simulink model "SF045A_HwAgSysArbn"  (R2013b)
settings: Solver=FixedStepDiscrete  SolverMode=SingleTasking  StartTime=0.0  StopTime=1  FixedStep=.002  RelTol=1e-3
values from neighbouring files (symbols this model uses):
  ARCHGLBPRM_2MILLISEC_SEC_F32 = DataDict.Constant    [SF045A_HwAgSysArbn_DataDict.m]
  ARCHGLBPRM_FLOATZEROTHD_ULS_F32 = DataDict.Constant    [SF045A_HwAgSysArbn_DataDict.m]
  ARCHGLBPRM_PIOVER180_ULS_F32 = DataDict.Constant    [SF045A_HwAgSysArbn_DataDict.m]
  CNVSECTOCNT_ULS_U32 = DataDict.Constant    [SF045A_HwAgSysArbn_DataDict.m]
  CNVTOMILLISEC_MILLISECPERCNT_F32 = DataDict.Constant    [SF045A_HwAgSysArbn_DataDict.m]
  FltInj_f32 = DataDict.Client    [SF045A_HwAgSysArbn_DataDict.m]
  FLTINJ_HWAGSYSARBN_HWAG = DataDict.Constant    [SF045A_HwAgSysArbn_DataDict.m]
  FLTINJ_HWAGSYSARBN_SERLCOMHWAG = DataDict.Constant    [SF045A_HwAgSysArbn_DataDict.m]
  HwAgCorrlnFlt = DataDict.NTC    [SF045A_HwAgSysArbn_DataDict.m]
  HwAgSnsrlsThdExcdd = DataDict.NTC    [SF045A_HwAgSysArbn_DataDict.m]
  HwAgSysArbnHwAgConf1Snsr = DataDict.Calibration    [SF045A_HwAgSysArbn_DataDict.m]
  HwAgSysArbnHwAgConf2Snsr = DataDict.Calibration    [SF045A_HwAgSysArbn_DataDict.m]
  HwAgSysArbnHwAgConfNoSnsr = DataDict.Calibration    [SF045A_HwAgSysArbn_DataDict.m]
  HwAgSysArbnHwAgCorrdCorrlnThd = DataDict.Calibration    [SF045A_HwAgSysArbn_DataDict.m]
  HwAgSysArbnHwAgCorrlnFailDebStep = DataDict.Calibration    [SF045A_HwAgSysArbn_DataDict.m]
  HwAgSysArbnHwAgCorrlnPassDebStep = DataDict.Calibration    [SF045A_HwAgSysArbn_DataDict.m]
  HwAgSysArbnHwAgCorrlnRng = DataDict.Calibration    [SF045A_HwAgSysArbn_DataDict.m]
  HwAgSysArbnHwAgSlewRate = DataDict.Calibration    [SF045A_HwAgSysArbn_DataDict.m]
  HwAgSysArbnHwAgSnsrlsCorrlnThd = DataDict.Calibration    [SF045A_HwAgSysArbn_DataDict.m]
  HwAgSysArbnHwAgSnsrlsKineThd = DataDict.Calibration    [SF045A_HwAgSysArbn_DataDict.m]
  HwAgSysArbnHwAgToMotAgCorrlnElpdTiLim = DataDict.Calibration    [SF045A_HwAgSysArbn_DataDict.m]
  HwAgSysArbnSerlComHwAgCorrdConf = DataDict.Calibration    [SF045A_HwAgSysArbn_DataDict.m]
  HwAgSysArbnSerlComHwAgSnsrlsConf = DataDict.Calibration    [SF045A_HwAgSysArbn_DataDict.m]
  HwAgSysArbnSlewRateTmr = DataDict.Calibration    [SF045A_HwAgSysArbn_DataDict.m]
  HWAGTHD_ULS_FLOAT32 = DataDict.Constant    [SF045A_HwAgSysArbn_DataDict.m]
  INVLDSRC_CNT_S08 = DataDict.Constant    [SF045A_HwAgSysArbn_DataDict.m]
  LRGSLEW_HWDEGPERSEC_F32 = DataDict.Constant    [SF045A_HwAgSysArbn_DataDict.m]
  NODEBSTEP_CNT_U16 = DataDict.Constant    [SF045A_HwAgSysArbn_DataDict.m]
  SLEWINPROGS_CNT_LGC = DataDict.Constant    [SF045A_HwAgSysArbn_DataDict.m]
  SLEWNOTINPROGS_CNT_LGC = DataDict.Constant    [SF045A_HwAgSysArbn_DataDict.m]
  SNSRDATASRCSELD_CNT_S08 = DataDict.Constant    [SF045A_HwAgSysArbn_DataDict.m]
  SNSRLSDATASRCSELD_CNT_S08 = DataDict.Constant    [SF045A_HwAgSysArbn_DataDict.m]
  SysGlbPrmSysKineRat = DataDict.ImprtdCal    [SF045A_HwAgSysArbn_DataDict.m]
  SysGlbPrmTorsBarStfn = DataDict.ImprtdCal    [SF045A_HwAgSysArbn_DataDict.m]
  ZEROTMR_MILLISEC_F32 = DataDict.Constant    [SF045A_HwAgSysArbn_DataDict.m]
undefined symbols (not defined in the file or in its folder): NtcSts1
libraries: NxtrLim x11, simulink x6, NxtrAbslt x6, Fil x3, autosarlib x2
(part 5 of 6)

== system SF045A_HwAgSysArbn/HwAgSysArbn/HwAgSysArbnPer1/HwAgArbn/CalcPinionVel/PinionAnglegConf/HwAg_Derivative ==
  HwAg : Inport
  Add2 : Sum  RequirementInfo="{'linktype_rmi_doors' '00012ce0 (/E-STEER Core/SubSystem Specifications/Application Functions - EA4/SF045A Handwheel Angle System Arbitration)' '#SF045A_139' 'true' 'REQ:  SF045A_139' '' } %GIDa_72753136_d011_4c3e_a530_2b55dc32ccf8"  Inputs=+-
  Constant1 : Constant  RequirementInfo="{'linktype_rmi_doors' '00012ce0 (/E-STEER Core/SubSystem Specifications/Application Functions - EA4/SF045A Handwheel Angle System Arbitration)' '#SF045A_139' 'true' 'REQ:  SF045A_139' '' } %GIDa_27737f0a_30e3_4100_8d18_fa88f0d6b124"  Value=ARCHGLBPRM_PIOVER180_ULS_F32
  CopyRight2 : Subsystem  Description=|  mask(Copyright Information){none=on}
      | Copyright info block.                                               
      |                                                                     
      | Place copyright information at the top of every subsystem in design.
      mask prompts: none "No parameters"
      mask help: Place copyright information at the top of every subsystem in design.
      mask Display:
      | NxtrConf = 'Nexteer Confidential';
      | 
      | sys = bdroot; %handle for the current model ("system")
      | first = get_param(sys,'Created');
      | first = first(end-3:end);  %year is last four digits
      | 
      | last = get_param(sys,'LastModifiedDate');
      | if isempty(last)
      |     last = datestr(now,'yyyy');
      | else
      |     last = last(end-3:end);
      | end
      | 
      | if strcmp(first,last)
      |     fprintf('%s -- Copyright %s Nexteer',NxtrConf,first)
      | else
      |     fprintf('%s -- %s%s- %s Nexteer',NxtrConf,char(169),first,last)
      | end
  Data Store Read : DataStoreRead  RequirementInfo="{'linktype_rmi_doors' '00012ce0 (/E-STEER Core/SubSystem Specifications/Application Functions - EA4/SF045A Handwheel Angle System Arbitration)' '#SF045A_139' 'true' 'REQ:  SF045A_139' '' } %GIDa_6b8d296a_e1fc_4324_90da_d5a7e0cde821"  Priority=1  DataStoreName=HwAgPrev
      settings: AttributesFormatString=Priority%<priority>
  Data Store Write : DataStoreWrite  RequirementInfo="{'linktype_rmi_doors' '00012ce0 (/E-STEER Core/SubSystem Specifications/Application Functions - EA4/SF045A Handwheel Angle System Arbitration)' '#SF045A_139' 'true' 'REQ:  SF045A_139' '' } %GIDa_6c16deaa_ea6f_4148_bb47_f580a11ebc09"  Priority=2  DataStoreName=HwAgPrev
      settings: AttributesFormatString=priority %<Priority>
  Divide1 : Product  RequirementInfo="{'linktype_rmi_doors' '00012ce0 (/E-STEER Core/SubSystem Specifications/Application Functions - EA4/SF045A Handwheel Angle System Arbitration)' '#SF045A_139' 'true' 'REQ:  SF045A_139' '' } %GIDa_8a642d90_b2e2_4998_af7d_68e21f55f73d"  Inputs=*/
  LoopTime1 : Constant  RequirementInfo="{'linktype_rmi_doors' '00012ce0 (/E-STEER Core/SubSystem Specifications/Application Functions - EA4/SF045A Handwheel Angle System Arbitration)' '#SF045A_139' 'true' 'REQ:  SF045A_139' '' } %GIDa_2a82eab3_347d_42e5_85a9_f87cdc562366"  Value=ARCHGLBPRM_2MILLISEC_SEC_F32
  Mult2 : Product  RequirementInfo="{'linktype_rmi_doors' '00012ce0 (/E-STEER Core/SubSystem Specifications/Application Functions - EA4/SF045A Handwheel Angle System Arbitration)' '#SF045A_139' 'true' 'REQ:  SF045A_139' '' } %GIDa_cfefcb1c_46ab_4711_9834_9b9f2488c419"  Inputs=**
  HwAg_Der : Outport
  wires:
  HwAg/1 -> Data Store Write/1, Add2/1
  Data Store Read/1 -> Add2/2
  Divide1/1 -> Mult2/1
  Add2/1 -> Divide1/1
  LoopTime1/1 -> Divide1/2
  Constant1/1 -> Mult2/2
  Mult2/1 -> HwAg_Der/1

== system SF045A_HwAgSysArbn/HwAgSysArbn/HwAgSysArbnPer1/HwAgArbn/CalcPinionVel/PinionAnglegConf/TbarVelocity ==
  HwTq : Inport  RequirementInfo={} %GIDa_c4b869cb_1139_4e42_8e94_0d7470ddf701
  Add2 : Sum  RequirementInfo="{'linktype_rmi_doors' '00012ce0 (/E-STEER Core/SubSystem Specifications/Application Functions - EA4/SF045A Handwheel Angle System Arbitration)' '#SF045A_137' 'true' 'REQ:  SF045A_137' '' } %GIDa_d4d3a053_9ce4_483a_97d0_fc540739ff80"  Inputs=+-
  Constant1 : Constant  RequirementInfo="{'linktype_rmi_doors' '00012ce0 (/E-STEER Core/SubSystem Specifications/Application Functions - EA4/SF045A Handwheel Angle System Arbitration)' '#SF045A_137' 'true' 'REQ:  SF045A_137' '' } %GIDa_2f4ecdc3_157e_4a87_a767_f147ebf34a5d"  Value=ARCHGLBPRM_PIOVER180_ULS_F32
  CopyRight2 : Subsystem  Description=|  mask(Copyright Information){none=on}
      | Copyright info block.                                               
      |                                                                     
      | Place copyright information at the top of every subsystem in design.
      mask prompts: none "No parameters"
      mask help: Place copyright information at the top of every subsystem in design.
      mask Display:
      | NxtrConf = 'Nexteer Confidential';
      | 
      | sys = bdroot; %handle for the current model ("system")
      | first = get_param(sys,'Created');
      | first = first(end-3:end);  %year is last four digits
      | 
      | last = get_param(sys,'LastModifiedDate');
      | if isempty(last)
      |     last = datestr(now,'yyyy');
      | else
      |     last = last(end-3:end);
      | end
      | 
      | if strcmp(first,last)
      |     fprintf('%s -- Copyright %s Nexteer',NxtrConf,first)
      | else
      |     fprintf('%s -- %s%s- %s Nexteer',NxtrConf,char(169),first,last)
      | end
  Data Store Read : DataStoreRead  RequirementInfo="{'linktype_rmi_doors' '00012ce0 (/E-STEER Core/SubSystem Specifications/Application Functions - EA4/SF045A Handwheel Angle System Arbitration)' '#SF045A_137' 'true' 'REQ:  SF045A_137' '' } %GIDa_284cc7a7_eefd_46a6_b2fe_8c7e1a0a81dd"  Priority=1  DataStoreName=TqSnsrAgPrev
      settings: AttributesFormatString=Priority%<priority>
  Data Store Write : DataStoreWrite  RequirementInfo="{'linktype_rmi_doors' '00012ce0 (/E-STEER Core/SubSystem Specifications/Application Functions - EA4/SF045A Handwheel Angle System Arbitration)' '#SF045A_137' 'true' 'REQ:  SF045A_137' '' } %GIDa_877a1179_72bf_41aa_b01f_35b294baab35"  Priority=2  DataStoreName=TqSnsrAgPrev
      settings: AttributesFormatString=priority %<Priority>
  Divide : Product  RequirementInfo="{'linktype_rmi_doors' '00012ce0 (/E-STEER Core/SubSystem Specifications/Application Functions - EA4/SF045A Handwheel Angle System Arbitration)' '#SF045A_137' 'true' 'REQ:  SF045A_137' '' } %GIDa_8a28dc6f_baa5_4599_acda_56322c814f34"  Inputs=*/
  Divide1 : Product  RequirementInfo="{'linktype_rmi_doors' '00012ce0 (/E-STEER Core/SubSystem Specifications/Application Functions - EA4/SF045A Handwheel Angle System Arbitration)' '#SF045A_137' 'true' 'REQ:  SF045A_137' '' } %GIDa_8d4da0b5_6a8d_47db_bb3c_04d8f790397b"  Inputs=*/
  FilLpUpdOutp : Fil/FilLpUpdOutp  RequirementInfo="{'linktype_rmi_doors' '00012ce0 (/E-STEER Core/SubSystem Specifications/Application Functions - EA4/SF045A Handwheel Angle System Arbitration)' '#SF045A_137' 'true' 'REQ:  SF045A_137' '' } %GIDa_6286290f_9601_4d52_893e_d57d1a2716fe"  StVar=TqSnsrVelFil
      settings: AttributesFormatString=StVar: %<StVar>
  LoopTime1 : Constant  RequirementInfo="{'linktype_rmi_doors' '00012ce0 (/E-STEER Core/SubSystem Specifications/Application Functions - EA4/SF045A Handwheel Angle System Arbitration)' '#SF045A_137' 'true' 'REQ:  SF045A_137' '' } %GIDa_143b2eb9_2257_4233_9d32_ab10b8cbc7a4"  Value=ARCHGLBPRM_2MILLISEC_SEC_F32
  Mult2 : Product  RequirementInfo="{'linktype_rmi_doors' '00012ce0 (/E-STEER Core/SubSystem Specifications/Application Functions - EA4/SF045A Handwheel Angle System Arbitration)' '#SF045A_137' 'true' 'REQ:  SF045A_137' '' } %GIDa_21c86b97_821a_4301_a3b3_2be767b326ad"  Inputs=**
  k_S_TbarStiff_NmpDeg_u9p7 : Constant  RequirementInfo="{'linktype_rmi_doors' '00012ce0 (/E-STEER Core/SubSystem Specifications/Application Functions - EA4/SF045A Handwheel Angle System Arbitration)' '#SF045A_137' 'true' 'REQ:  SF045A_137' '' } %GIDa_b6c06969_045a_4d51_9719_dc8d98d8c8a3"  Value=SysGlbPrmTorsBarStfn
  TbarVel : Outport
  wires:
  HwTq/1 -> Divide/1
  k_S_TbarStiff_NmpDeg_u9p7/1 -> Divide/2
  Divide/1 -> Add2/1, Data Store Write/1
  Divide1/1 -> FilLpUpdOutp/1
  FilLpUpdOutp/1 -> Mult2/1
  Add2/1 -> Divide1/1
  LoopTime1/1 -> Divide1/2
  Data Store Read/1 -> Add2/2
  Constant1/1 -> Mult2/2
  Mult2/1 -> TbarVel/1  "TbarVel_HwRadPerSec_T_f32"

== system SF045A_HwAgSysArbn/HwAgSysArbn/HwAgSysArbnPer1/HwAgArbn/CalcPinionVel/ZeroState/CopyRight2 ==

== system SF045A_HwAgSysArbn/HwAgSysArbn/HwAgSysArbnPer1/HwAgArbn/HwAgSrcSeln/SnsrlsHwAgSeln/CopyRight2 ==

== system SF045A_HwAgSysArbn/HwAgSysArbn/HwAgSysArbnPer1/HwAgArbn/HwAgSrcSeln/VrfyHwAgCorrln/CopyRight2 ==

== system SF045A_HwAgSysArbn/HwAgSysArbn/HwAgSysArbnPer1/HwAgArbn/HwAgSrcSeln/VrfyHwAgCorrln/HwAgCorrdConfCalc ==
  HwAgCorrdConf : Inport
  Action Port : ActionPort  ActionType=then
  CopyRight2 : Subsystem  Description=|  mask(Copyright Information){none=on}
      | Copyright info block.                                               
      |                                                                     
      | Place copyright information at the top of every subsystem in design.
      mask prompts: none "No parameters"
      mask help: Place copyright information at the top of every subsystem in design.
      mask Display:
      | NxtrConf = 'Nexteer Confidential';
      | 
      | sys = bdroot; %handle for the current model ("system")
      | first = get_param(sys,'Created');
      | first = first(end-3:end);  %year is last four digits
      | 
      | last = get_param(sys,'LastModifiedDate');
      | if isempty(last)
      |     last = datestr(now,'yyyy');
      | else
      |     last = last(end-3:end);
      | end
      | 
      | if strcmp(first,last)
      |     fprintf('%s -- Copyright %s Nexteer',NxtrConf,first)
      | else
      |     fprintf('%s -- %s%s- %s Nexteer',NxtrConf,char(169),first,last)
      | end
  HwAgConf : Outport
  wires:
  HwAgCorrdConf/1 -> HwAgConf/1

== system SF045A_HwAgSysArbn/HwAgSysArbn/HwAgSysArbnPer1/HwAgArbn/HwAgSrcSeln/VrfyHwAgCorrln/HwAgCorrdLatch ==
  HwAgCorrd : Inport
  Action Port : ActionPort  ActionType=then
  Abslt_f32_f3 : NxtrAbslt/Abslt_f32_f32  RequirementInfo={} %GIDa_74010d29_d7b0_454c_872f_0f7019f095ef  SFunctionSpec=single y1 = Abslt_f32_f32(single u1)
      settings: AttributesFormatString=%<Name>
  Constant4 : Constant  RequirementInfo={} %GIDa_f84fbda8_7081_4bb5_be38_89aa74422cd7  Value=ARCHGLBPRM_FLOATZEROTHD_ULS_F32
  CopyRight2 : Subsystem  Description=|  mask(Copyright Information){none=on}
      | Copyright info block.                                               
      |                                                                     
      | Place copyright information at the top of every subsystem in design.
      mask prompts: none "No parameters"
      mask help: Place copyright information at the top of every subsystem in design.
      mask Display:
      | NxtrConf = 'Nexteer Confidential';
      | 
      | sys = bdroot; %handle for the current model ("system")
      | first = get_param(sys,'Created');
      | first = first(end-3:end);  %year is last four digits
      | 
      | last = get_param(sys,'LastModifiedDate');
      | if isempty(last)
      |     last = datestr(now,'yyyy');
      | else
      |     last = last(end-3:end);
      | end
      | 
      | if strcmp(first,last)
      |     fprintf('%s -- Copyright %s Nexteer',NxtrConf,first)
      | else
      |     fprintf('%s -- %s%s- %s Nexteer',NxtrConf,char(169),first,last)
      | end
  Data Store Write : DataStoreWrite  RequirementInfo="{'linktype_rmi_doors' '00012ce0 (/E-STEER Core/SubSystem Specifications/Application Functions - EA4/SF045A Handwheel Angle System Arbitration)' '#SF045A_137' 'true' 'REQ:  SF045A_137' '' } %GIDa_3f417201_3964_4138_9f7e_764d42d6c10e"  Priority=2  DataStoreName=HwAgCorrdLtch
      settings: AttributesFormatString=Priority%<priority>
  Relational Operator5 : RelationalOperator  RequirementInfo={} %GIDa_78acdf02_6e94_4055_ad37_114f5c0d7fb0  Operator=>  OutDataTypeStr=boolean
  wires:
  HwAgCorrd/1 -> Abslt_f32_f3/1
  Constant4/1 -> Relational Operator5/2
  Abslt_f32_f3/1 -> Relational Operator5/1
  Relational Operator5/1 -> Data Store Write/1

== system SF045A_HwAgSysArbn/HwAgSysArbn/HwAgSysArbnPer1/HwAgArbn/HwAgSrcSeln/VrfyHwAgCorrln/ZeroStateAgCong ==
  Action Port : ActionPort  ActionType=else
  CopyRight2 : Subsystem  Description=|  mask(Copyright Information){none=on}
      | Copyright info block.                                               
      |                                                                     
      | Place copyright information at the top of every subsystem in design.
      mask prompts: none "No parameters"
      mask help: Place copyright information at the top of every subsystem in design.
      mask Display:
      | NxtrConf = 'Nexteer Confidential';
      | 
      | sys = bdroot; %handle for the current model ("system")
      | first = get_param(sys,'Created');
      | first = first(end-3:end);  %year is last four digits
      | 
      | last = get_param(sys,'LastModifiedDate');
      | if isempty(last)
      |     last = datestr(now,'yyyy');
      | else
      |     last = last(end-3:end);
      | end
      | 
      | if strcmp(first,last)
      |     fprintf('%s -- Copyright %s Nexteer',NxtrConf,first)
      | else
      |     fprintf('%s -- %s%s- %s Nexteer',NxtrConf,char(169),first,last)
      | end
  PinionVelConfFalse : Constant  Value=0  OutDataTypeStr=single
      settings: AttributesFormatString=%<OutDataTypeStr>
  FALSE_HwAgConf : Outport
  wires:
  PinionVelConfFalse/1 -> FALSE_HwAgConf/1

== system SF045A_HwAgSysArbn/HwAgSysArbn/HwAgSysArbnPer1/HwAgArbn/HwAgVelSeriCom/ChkCorrln/CopyRight2 ==

== system SF045A_HwAgSysArbn/HwAgSysArbn/HwAgSysArbnPer1/HwAgArbn/HwAgVelSeriCom/ChkCorrln/SetCorrlFltNtc ==
  Action Port : ActionPort  ActionType=else
  Constant1 : Constant  RequirementInfo={} %GIDa_29c0768e_b7da_408e_a59c_493179b59f0b  Value=0
  Constant2 : Constant  RequirementInfo={} %GIDa_de5f8f58_792a_4fb2_a119_adcc623982ab  Value=HwAgSysArbnHwAgCorrlnFailDebStep
  Constant3 : Constant  RequirementInfo={} %GIDa_b4614c80_3746_4b05_a304_4c7fd58d9eae  Value=HwAgCorrlnFlt
  Constant4 : Constant  RequirementInfo={} %GIDa_66946ee4_abc4_4d82_825c_f9bc77a77541  Value=false  OutDataTypeStr=boolean
      settings: AttributesFormatString=%<OutDataTypeStr>
  CopyRight2 : Subsystem  Description=|  mask(Copyright Information){none=on}
      | Copyright info block.                                               
      |                                                                     
      | Place copyright information at the top of every subsystem in design.
      mask prompts: none "No parameters"
      mask help: Place copyright information at the top of every subsystem in design.
      mask Display:
      | NxtrConf = 'Nexteer Confidential';
      | 
      | sys = bdroot; %handle for the current model ("system")
      | first = get_param(sys,'Created');
      | first = first(end-3:end);  %year is last four digits
      | 
      | last = get_param(sys,'LastModifiedDate');
      | if isempty(last)
      |     last = datestr(now,'yyyy');
      | else
      |     last = last(end-3:end);
      | end
      | 
      | if strcmp(first,last)
      |     fprintf('%s -- Copyright %s Nexteer',NxtrConf,first)
      | else
      |     fprintf('%s -- %s%s- %s Nexteer',NxtrConf,char(169),first,last)
      | end
  Data Store Write1 : DataStoreWrite  RequirementInfo={} %GIDa_3f8d0d30_5fdb_4d6a_ae2a_ecaaf85c60f5  DataStoreName=HwAgToMotAgCorrln
  Enumerated Constant1 : simulink/Sources/Enumerated Constant  RequirementInfo={} %GIDa_fe4ef9a3_1e6d_4bc0_939b_dcc775b098ca  OutDataTypeStr=Enum: NtcSts1  Value=NtcSts1.NTCSTS_PREFAILD  SampleTime=inf
  SetCorrlFltNtc : Subsystem  RequirementInfo={} %GIDa_aeb47bce_6be1_4638_8e96_a2172e981274  mask(SetNTC){}
      mask help: SetNTC library block
  wires:
  Enumerated Constant1/1 -> SetCorrlFltNtc/3(NtcSts)
  Constant1/1 -> SetCorrlFltNtc/2(NtcStInfo)
  Constant3/1 -> SetCorrlFltNtc/1(NtcNr)
  Constant2/1 -> SetCorrlFltNtc/4(DebStep)
  Constant4/1 -> Data Store Write1/1

== system SF045A_HwAgSysArbn/HwAgSysArbn/HwAgSysArbnPer1/HwAgArbn/HwAgVelSeriCom/ChkCorrln/SetNtcPass ==
  Action Port : ActionPort  ActionType=then
  Constant15 : Constant  RequirementInfo={} %GIDa_07d87f94_c688_4e33_a636_a79e35048b97  Value=HwAgSysArbnHwAgCorrlnPassDebStep
  Constant18 : Constant  RequirementInfo={} %GIDa_7f55d612_ca22_4677_b2c1_49008eac2b51  Value=0
  Constant3 : Constant  RequirementInfo={} %GIDa_b89e6fbd_b50e_42d4_8bea_9bfa1c5ebf24  Value=HwAgCorrlnFlt
  Constant4 : Constant  RequirementInfo={} %GIDa_0265ae9f_aeb8_4b58_8f74_dcd9ec1ca95e  Value=true  OutDataTypeStr=boolean
      settings: AttributesFormatString=%<OutDataTypeStr>
  CopyRight2 : Subsystem  Description=|  mask(Copyright Information){none=on}
      | Copyright info block.                                               
      |                                                                     
      | Place copyright information at the top of every subsystem in design.
      mask prompts: none "No parameters"
      mask help: Place copyright information at the top of every subsystem in design.
      mask Display:
      | NxtrConf = 'Nexteer Confidential';
      | 
      | sys = bdroot; %handle for the current model ("system")
      | first = get_param(sys,'Created');
      | first = first(end-3:end);  %year is last four digits
      | 
      | last = get_param(sys,'LastModifiedDate');
      | if isempty(last)
      |     last = datestr(now,'yyyy');
      | else
      |     last = last(end-3:end);
      | end
      | 
      | if strcmp(first,last)
      |     fprintf('%s -- Copyright %s Nexteer',NxtrConf,first)
      | else
      |     fprintf('%s -- %s%s- %s Nexteer',NxtrConf,char(169),first,last)
      | end
  Data Store Write1 : DataStoreWrite  RequirementInfo={} %GIDa_de7e9dca_d214_4286_8c42_bc77e497324a  DataStoreName=HwAgToMotAgCorrlnDurnRefTmr
  Data Store Write3 : DataStoreWrite  RequirementInfo={} %GIDa_466ac138_7d86_4ee8_8614_c84b2fb52692  DataStoreName=HwAgToMotAgCorrln
  Enumerated Constant13 : simulink/Sources/Enumerated Constant  RequirementInfo={} %GIDa_43e7e443_2a05_417e_9e96_9af6d500f356  OutDataTypeStr=Enum: NtcSts1  Value=NtcSts1.NTCSTS_PREPASSD  SampleTime=inf
  GetRefTmr100MicroSec32bit : Subsystem  RequirementInfo={} %GIDa_66d8492a_abb8_4461_bb12_8703988925df
  SetNtcPass : Subsystem  RequirementInfo={} %GIDa_b1c204ca_8313_42a8_80eb_f2e70d60a35d  mask(SetNTC){}
      mask help: SetNTC library block
  wires:
  Constant15/1 -> SetNtcPass/4(DebStep)
  Enumerated Constant13/1 -> SetNtcPass/3(NtcSts)
  Constant18/1 -> SetNtcPass/2(NtcStInfo)
  Constant3/1 -> SetNtcPass/1(NtcNr)
  Constant4/1 -> Data Store Write3/1
  GetRefTmr100MicroSec32bit/1(RefTmr) -> Data Store Write1/1

== system SF045A_HwAgSysArbn/HwAgSysArbn/HwAgSysArbnPer1/HwAgArbn/HwAgVelSeriCom/NoHwAgDataToSerlCom/CopyRight2 ==

== system SF045A_HwAgSysArbn/HwAgSysArbn/HwAgSysArbnPer1/HwAgArbn/HwAgVelSeriCom/SnsrDataToSerlCom/CopyRight2 ==

== system SF045A_HwAgSysArbn/HwAgSysArbn/HwAgSysArbnPer1/HwAgArbn/HwAgVelSeriCom/SnsrlsDataToSerlCom/CopyRight2 ==

== system SF045A_HwAgSysArbn/HwAgSysArbn/HwAgSysArbnPer1/HwAgArbn/HwAgVelSeriCom/SnsrlsDataToSerlCom/CorrlnStsFalse ==
  Action Port : ActionPort  ActionType=else
  Constant1 : Constant  RequirementInfo={} %GIDa_a9405739_f3c9_4238_b8c8_f50b6ead1583  Value=0  OutDataTypeStr=single
      settings: AttributesFormatString=%<OutDataTypeStr>
  Constant3 : Constant  RequirementInfo={} %GIDa_f17cf790_4675_4924_b51f_aa5a8df77093  Value=0  OutDataTypeStr=boolean
      settings: AttributesFormatString=%<OutDataTypeStr>
  CopyRight2 : Subsystem  Description=|  mask(Copyright Information){none=on}
      | Copyright info block.                                               
      |                                                                     
      | Place copyright information at the top of every subsystem in design.
      mask prompts: none "No parameters"
      mask help: Place copyright information at the top of every subsystem in design.
      mask Display:
      | NxtrConf = 'Nexteer Confidential';
      | 
      | sys = bdroot; %handle for the current model ("system")
      | first = get_param(sys,'Created');
      | first = first(end-3:end);  %year is last four digits
      | 
      | last = get_param(sys,'LastModifiedDate');
      | if isempty(last)
      |     last = datestr(now,'yyyy');
      | else
      |     last = last(end-3:end);
      | end
      | 
      | if strcmp(first,last)
      |     fprintf('%s -- Copyright %s Nexteer',NxtrConf,first)
      | else
      |     fprintf('%s -- %s%s- %s Nexteer',NxtrConf,char(169),first,last)
      | end
  HwAgToSerlCom : Outport  RequirementInfo={} %GIDa_84de3b2f_036e_414c_a20a_e4321f550f97
  HwAgStsToSerlCom : Outport  RequirementInfo={} %GIDa_0df8a081_101b_4dd2_873f_2f2cc18236ee  Port=2
  wires:
  Constant3/1 -> HwAgStsToSerlCom/1
  Constant1/1 -> HwAgToSerlCom/1

== system SF045A_HwAgSysArbn/HwAgSysArbn/HwAgSysArbnPer1/HwAgArbn/HwAgVelSeriCom/SnsrlsDataToSerlCom/CorrlnStsTrue ==
  HwAgSnsrls : Inport
  HwAgSnsrlsConf : Inport  Port=2
  Action Port : ActionPort  ActionType=then
  Constant8 : Constant  RequirementInfo={} %GIDa_fb4632ee_8ffa_4ef4_822a_201cfbcc10ac  Value=HwAgSysArbnSerlComHwAgSnsrlsConf
  CopyRight2 : Subsystem  Description=|  mask(Copyright Information){none=on}
      | Copyright info block.                                               
      |                                                                     
      | Place copyright information at the top of every subsystem in design.
      mask prompts: none "No parameters"
      mask help: Place copyright information at the top of every subsystem in design.
      mask Display:
      | NxtrConf = 'Nexteer Confidential';
      | 
      | sys = bdroot; %handle for the current model ("system")
      | first = get_param(sys,'Created');
      | first = first(end-3:end);  %year is last four digits
      | 
      | last = get_param(sys,'LastModifiedDate');
      | if isempty(last)
      |     last = datestr(now,'yyyy');
      | else
      |     last = last(end-3:end);
      | end
      | 
      | if strcmp(first,last)
      |     fprintf('%s -- Copyright %s Nexteer',NxtrConf,first)
      | else
      |     fprintf('%s -- %s%s- %s Nexteer',NxtrConf,char(169),first,last)
      | end
  Relational Operator : RelationalOperator  RequirementInfo="{'linktype_rmi_doors' '00012ce0 (/E-STEER Core/SubSystem Specifications/Application Functions - EA4/SF045A Handwheel Angle System Arbitration)' '#SF045A_126' 'true' 'REQ:  SF045A_126' '' } %GIDa_2df6559f_4c97_46e3_a5cb_d6b8ab37a51a"  OutDataTypeStr=boolean
  HwAgToSerlCom : Outport
  HwAgStsToSerlCom : Outport  Port=2
  wires:
  Relational Operator/1 -> HwAgStsToSerlCom/1
  Constant8/1 -> Relational Operator/2
  HwAgSnsrlsConf/1 -> Relational Operator/1
  HwAgSnsrls/1 -> HwAgToSerlCom/1

== system SF045A_HwAgSysArbn/HwAgSysArbn/HwAgSysArbnPer1/HwAgArbn/HwAgVelSeriCom/SnsrlsDataToSerlCom/GetTiSpan100MicroSec32bit ==
  note: Created Aug 18, 2015
      | Modified Oct 21, 2015
      | Modified Oct 30, 2015
      | Kevin Derry
  note: GetTiSpan100MicroSec32bit
  note: Get current system time
  note: 1 count = 100 uSec
  note: Wrap-to-zero
  note: counts
  note: microseconds
  note: seconds
  note: Subtract original reference time
  RefTmr : Inport
  CopyRight2 : Subsystem  Description=|  mask(Copyright Information){none=on}
      | Copyright info block.                                               
      |                                                                     
      | Place copyright information at the top of every subsystem in design.
      mask prompts: none "No parameters"
      mask help: Place copyright information at the top of every subsystem in design.
      mask Display:
      | NxtrConf = 'Nexteer Confidential';
      | 
      | sys = bdroot; %handle for the current model ("system")
      | first = get_param(sys,'Created');
      | if(isempty(first))
      |     first = datestr(now,'yyyy');
      | else
      |     first = first(end-3:end);  %year is last four digits
      | end
      | 
      | last = get_param(sys,'LastModifiedDate');
      | if isempty(last)
      |     last = datestr(now,'yyyy');
      | else
      |     last = last(end-3:end);
      | end
      | 
      | if strcmp(first,last)
      |     fprintf('%s -- Copyright %s Nexteer',NxtrConf,first)
      | else
      |     fprintf('%s -- %s%s- %s Nexteer',NxtrConf,char(169),first,last)
      | end
  Count per uSec : Constant  Value=0.01
  Data Store Read1 : DataStoreRead  DataStoreName=SimnTi
  Data Type Conversion2 : DataTypeConversion  OutDataTypeStr=uint32
  Divide1 : Product  Inputs=**
  Divide2 : Product  Inputs=*/
  If : If  NumInputs=2  IfExpression=u1 >= u2
  Max Counts : Constant  Value=2^32-1
  Merge : Merge
  No wrapping : Subsystem  TreatAsAtomicUnit=on
  Product2 : Product
  Product3 : Product
  Rounding : Rounding
  Subtract3 : Sum  Inputs=+-
  Wrapping : Subsystem  TreatAsAtomicUnit=on
  uSec per Sec : Constant  Value=1000000
  TiSpan : Outport
  wires:
  Data Type Conversion2/1 -> Wrapping/1(new), No wrapping/1(new), If/1
  RefTmr/1 -> Wrapping/2(ref), No wrapping/2(ref), If/2
  Merge/1 -> TiSpan/1
  uSec per Sec/1 -> Product2/2
  Count per uSec/1 -> Divide1/2
  Data Store Read1/1 -> Product2/1
  Product2/1 -> Divide1/1
  Divide1/1 -> Subtract3/1, Divide2/1
  Max Counts/1 -> Product3/2, Divide2/2
  Divide2/1 -> Rounding/1
  Rounding/1 -> Product3/1
  Subtract3/1 -> Data Type Conversion2/1
  Product3/1 -> Subtract3/2
  If/1 -> No wrapping/Action
  If/2 -> Wrapping/Action
  No wrapping/1(Out1) -> Merge/1
  Wrapping/1(Out1) -> Merge/2

== system SF045A_HwAgSysArbn/HwAgSysArbn/HwAgSysArbnPer1/HwAgArbn/TestHwAgSrcChg/ApplyLrgSlew/CopyRight2 ==

== system SF045A_HwAgSysArbn/HwAgSysArbn/HwAgSysArbnPer1/HwAgArbn/TestHwAgSrcChg/ApplyRateLim/CopyRight2 ==

== system SF045A_HwAgSysArbn/HwAgSysArbn/HwAgSysArbnPer1/HwAgArbn/TestHwAgSrcChg/ApplyRateLim/GetTiSpan100MicroSec32bit ==
  note: Created Aug 18, 2015
      | Modified Oct 21, 2015
      | Modified Oct 30, 2015
      | Kevin Derry
  note: GetTiSpan100MicroSec32bit
  note: Get current system time
  note: 1 count = 100 uSec
  note: Wrap-to-zero
  note: counts
  note: microseconds
  note: seconds
  note: Subtract original reference time
  RefTmr : Inport
  CopyRight2 : Subsystem  Description=|  mask(Copyright Information){none=on}
      | Copyright info block.                                               
      |                                                                     
      | Place copyright information at the top of every subsystem in design.
      mask prompts: none "No parameters"
      mask help: Place copyright information at the top of every subsystem in design.
      mask Display:
      | NxtrConf = 'Nexteer Confidential';
      | 
      | sys = bdroot; %handle for the current model ("system")
      | first = get_param(sys,'Created');
      | if(isempty(first))
      |     first = datestr(now,'yyyy');
      | else
      |     first = first(end-3:end);  %year is last four digits
      | end
      | 
      | last = get_param(sys,'LastModifiedDate');
      | if isempty(last)
      |     last = datestr(now,'yyyy');
      | else
      |     last = last(end-3:end);
      | end
      | 
      | if strcmp(first,last)
      |     fprintf('%s -- Copyright %s Nexteer',NxtrConf,first)
      | else
      |     fprintf('%s -- %s%s- %s Nexteer',NxtrConf,char(169),first,last)
      | end
  Count per uSec : Constant  Value=0.01
  Data Store Read1 : DataStoreRead  DataStoreName=SimnTi
  Data Type Conversion2 : DataTypeConversion  OutDataTypeStr=uint32
  Divide1 : Product  Inputs=**
  Divide2 : Product  Inputs=*/
  If : If  NumInputs=2  IfExpression=u1 >= u2
  Max Counts : Constant  Value=2^32-1
  Merge : Merge
  No wrapping : Subsystem  TreatAsAtomicUnit=on
  Product2 : Product
  Product3 : Product
  Rounding : Rounding
  Subtract3 : Sum  Inputs=+-
  Wrapping : Subsystem  TreatAsAtomicUnit=on
  uSec per Sec : Constant  Value=1000000
  TiSpan : Outport
  wires:
  Data Type Conversion2/1 -> Wrapping/1(new), No wrapping/1(new), If/1
  RefTmr/1 -> Wrapping/2(ref), No wrapping/2(ref), If/2
  Merge/1 -> TiSpan/1
  uSec per Sec/1 -> Product2/2
  Count per uSec/1 -> Divide1/2
  Data Store Read1/1 -> Product2/1
  Product2/1 -> Divide1/1
  Divide1/1 -> Subtract3/1, Divide2/1
  Max Counts/1 -> Product3/2, Divide2/2
  Divide2/1 -> Rounding/1
  Rounding/1 -> Product3/1
  Subtract3/1 -> Data Type Conversion2/1
  Product3/1 -> Subtract3/2
  If/1 -> No wrapping/Action
  If/2 -> Wrapping/Action
  No wrapping/1(Out1) -> Merge/1
  Wrapping/1(Out1) -> Merge/2

== system SF045A_HwAgSysArbn/HwAgSysArbn/HwAgSysArbnPer1/HwAgArbn/TestHwAgSrcChg/ApplyRateLim/Pass ==
  note: Pass on the computed values of Hw Ag Confidence as Slewing is not in progress
  HwAgConfInp : Inport
  Action Port : ActionPort  ActionType=else
  Constant4 : Constant  Value=SLEWNOTINPROGS_CNT_LGC
  CopyRight2 : Subsystem  Description=|  mask(Copyright Information){none=on}
      | Copyright info block.                                               
      |                                                                     
      | Place copyright information at the top of every subsystem in design.
      mask prompts: none "No parameters"
      mask help: Place copyright information at the top of every subsystem in design.
      mask Display:
      | NxtrConf = 'Nexteer Confidential';
      | 
      | sys = bdroot; %handle for the current model ("system")
      | first = get_param(sys,'Created');
      | first = first(end-3:end);  %year is last four digits
      | 
      | last = get_param(sys,'LastModifiedDate');
      | if isempty(last)
      |     last = datestr(now,'yyyy');
      | else
      |     last = last(end-3:end);
      | end
      | 
      | if strcmp(first,last)
      |     fprintf('%s -- Copyright %s Nexteer',NxtrConf,first)
      | else
      |     fprintf('%s -- %s%s- %s Nexteer',NxtrConf,char(169),first,last)
      | end
  Data Store Write5 : DataStoreWrite  RequirementInfo={} %GIDa_ecaac11c_55d7_4608_8542_e553c46da46d  DataStoreName=SlewSts
  "HwAgConf " : Outport
  wires:
  HwAgConfInp/1 -> "HwAgConf "/1
  Constant4/1 -> Data Store Write5/1

== system SF045A_HwAgSysArbn/HwAgSysArbn/HwAgSysArbnPer1/HwAgArbn/TestHwAgSrcChg/ApplyRateLim/RetainHwAgConf ==
  note: Pass on the previous values of Hw Ag Confidence as Slewing is not complete
  PrevHwAgConf : Inport
  Action Port : ActionPort  ActionType=then
  Constant4 : Constant  Value=SLEWINPROGS_CNT_LGC
  CopyRight2 : Subsystem  Description=|  mask(Copyright Information){none=on}
      | Copyright info block.                                               
      |                                                                     
      | Place copyright information at the top of every subsystem in design.
      mask prompts: none "No parameters"
      mask help: Place copyright information at the top of every subsystem in design.
      mask Display:
      | NxtrConf = 'Nexteer Confidential';
      | 
      | sys = bdroot; %handle for the current model ("system")
      | first = get_param(sys,'Created');
      | first = first(end-3:end);  %year is last four digits
      | 
      | last = get_param(sys,'LastModifiedDate');
      | if isempty(last)
      |     last = datestr(now,'yyyy');
      | else
      |     last = last(end-3:end);
      | end
      | 
      | if strcmp(first,last)
      |     fprintf('%s -- Copyright %s Nexteer',NxtrConf,first)
      | else
      |     fprintf('%s -- %s%s- %s Nexteer',NxtrConf,char(169),first,last)
      | end
  Data Store Write5 : DataStoreWrite  RequirementInfo={} %GIDa_c0913eba_fe2a_4ca0_81d7_48a13b0a077b  DataStoreName=SlewSts
  "HwAgConf " : Outport
  wires:
  PrevHwAgConf/1 -> "HwAgConf "/1
  Constant4/1 -> Data Store Write5/1

== system SF045A_HwAgSysArbn/HwAgSysArbn/HwAgSysArbnPer1/HwAgArbn/TestHwAgSrcChg/RetainSlewRate/CopyRight2 ==

== system SF045A_HwAgSysArbn/HwAgSysArbn/HwAgSysArbnPer1/HwAgArbn/TestHwAgSrcChg/SetSlewRate/CopyRight2 ==

== system SF045A_HwAgSysArbn/HwAgSysArbn/HwAgSysArbnPer1/HwAgArbn/TestHwAgSrcChg/SetSlewRate/GetRefTmr100MicroSec32bit ==
  note: 1 count = 100 uSec
  note: seconds
  note: microseconds
  note: counts
  note: Wrap-to-zero
  note: GetRefTmr100MicroSec32bit
  CopyRight2 : Subsystem  Description=|  mask(Copyright Information){none=on}
      | Copyright info block.                                               
      |                                                                     
      | Place copyright information at the top of every subsystem in design.
      mask prompts: none "No parameters"
      mask help: Place copyright information at the top of every subsystem in design.
      mask Display:
      | NxtrConf = 'Nexteer Confidential';
      | 
      | sys = bdroot; %handle for the current model ("system")
      | first = get_param(sys,'Created');
      | if(isempty(first))
      |     first = datestr(now,'yyyy');
      | else
      |     first = first(end-3:end);  %year is last four digits
      | end
      | 
      | last = get_param(sys,'LastModifiedDate');
      | if isempty(last)
      |     last = datestr(now,'yyyy');
      | else
      |     last = last(end-3:end);
      | end
      | 
      | if strcmp(first,last)
      |     fprintf('%s -- Copyright %s Nexteer',NxtrConf,first)
      | else
      |     fprintf('%s -- %s%s- %s Nexteer',NxtrConf,char(169),first,last)
      | end
  Count per uSec : Constant  Value=0.01
  Data Store Read1 : DataStoreRead  DataStoreName=SimnTi
  Data Type Conversion1 : DataTypeConversion  OutDataTypeStr=uint32
  Divide1 : Product  Inputs=**
  Divide2 : Product  Inputs=*/
  Max Counts : Constant  Value=2^32-1
  Product1 : Product
  Product2 : Product
  Rounding : Rounding
  Subtract1 : Sum  Inputs=+-
  uSec per Sec : Constant  Value=1000000
  RefTmr : Outport
  wires:
  Product2/1 -> Subtract1/2
  Subtract1/1 -> Data Type Conversion1/1
  Rounding/1 -> Product2/1
  Divide2/1 -> Rounding/1
  Max Counts/1 -> Divide2/2, Product2/2
  Divide1/1 -> Divide2/1, Subtract1/1
  Product1/1 -> Divide1/1
  Data Store Read1/1 -> Product1/1
  Count per uSec/1 -> Divide1/2
  uSec per Sec/1 -> Product1/2
  Data Type Conversion1/1 -> RefTmr/1

== system SF045A_HwAgSysArbn/HwAgSysArbn/HwAgSysArbnPer1/HwAgArbn/VldtSnsrlsData/Pass/CopyRight2 ==

== system SF045A_HwAgSysArbn/HwAgSysArbn/HwAgSysArbnPer1/HwAgArbn/VldtSnsrlsData/ThdExcdd/CopyRight2 ==

== system SF045A_HwAgSysArbn/HwAgSysArbn/HwAgSysArbnPer1/HwAgArbn/VldtSnsrlsData/ThdExcdd/Kinematic Integrity ==
  NtcNr : Inport
  NtcStInfo : Inport  Port=2
  NtcSts : Inport  Port=3
  DebStep : Inport  Port=4
  SetNtcSts : Subsystem  RequirementInfo={} %GIDa_0a4e7fc1_f133_4b51_96a9_40a2b0d33ec7  TreatAsAtomicUnit=on
      settings: RTWSystemCode=Inline
  wires:
  NtcStInfo/1 -> SetNtcSts/2(NtcStInfo)
  DebStep/1 -> SetNtcSts/4(DebStep)
  NtcSts/1 -> SetNtcSts/3(NtcSts)
  NtcNr/1 -> SetNtcSts/1(NtcNr)  "NtcNr"

== system SF045A_HwAgSysArbn/HwAgSysArbn/HwAgSysArbnPer1/HwAgArbn/CalcPinionVel/MotorVelocityVld/TbarVelocity/CopyRight2 ==

== system SF045A_HwAgSysArbn/HwAgSysArbn/HwAgSysArbnPer1/HwAgArbn/CalcPinionVel/PinionAnglegConf/HwAg_Derivative/CopyRight2 ==

== system SF045A_HwAgSysArbn/HwAgSysArbn/HwAgSysArbnPer1/HwAgArbn/CalcPinionVel/PinionAnglegConf/TbarVelocity/CopyRight2 ==

== system SF045A_HwAgSysArbn/HwAgSysArbn/HwAgSysArbnPer1/HwAgArbn/HwAgSrcSeln/VrfyHwAgCorrln/HwAgCorrdConfCalc/CopyRight2 ==

== system SF045A_HwAgSysArbn/HwAgSysArbn/HwAgSysArbnPer1/HwAgArbn/HwAgSrcSeln/VrfyHwAgCorrln/HwAgCorrdLatch/CopyRight2 ==

== system SF045A_HwAgSysArbn/HwAgSysArbn/HwAgSysArbnPer1/HwAgArbn/HwAgSrcSeln/VrfyHwAgCorrln/ZeroStateAgCong/CopyRight2 ==

== system SF045A_HwAgSysArbn/HwAgSysArbn/HwAgSysArbnPer1/HwAgArbn/HwAgVelSeriCom/ChkCorrln/SetCorrlFltNtc/CopyRight2 ==

== system SF045A_HwAgSysArbn/HwAgSysArbn/HwAgSysArbnPer1/HwAgArbn/HwAgVelSeriCom/ChkCorrln/SetCorrlFltNtc/SetCorrlFltNtc ==
  NtcNr : Inport
  NtcStInfo : Inport  Port=2
  NtcSts : Inport  Port=3
  DebStep : Inport  Port=4
  SetNtcSts : Subsystem  RequirementInfo={} %GIDa_090403ee_acf6_4527_bcbb_3b95fba33d1d  TreatAsAtomicUnit=on
      settings: RTWSystemCode=Inline
  wires:
  NtcStInfo/1 -> SetNtcSts/2(NtcStInfo)
  DebStep/1 -> SetNtcSts/4(DebStep)
  NtcSts/1 -> SetNtcSts/3(NtcSts)
  NtcNr/1 -> SetNtcSts/1(NtcNr)  "NtcNr"

== system SF045A_HwAgSysArbn/HwAgSysArbn/HwAgSysArbnPer1/HwAgArbn/HwAgVelSeriCom/ChkCorrln/SetNtcPass/CopyRight2 ==

== system SF045A_HwAgSysArbn/HwAgSysArbn/HwAgSysArbnPer1/HwAgArbn/HwAgVelSeriCom/ChkCorrln/SetNtcPass/GetRefTmr100MicroSec32bit ==
  note: 1 count = 100 uSec
  note: seconds
  note: microseconds
  note: counts
  note: Wrap-to-zero
  note: GetRefTmr100MicroSec32bit
  CopyRight2 : Subsystem  Description=|  mask(Copyright Information){none=on}
      | Copyright info block.                                               
      |                                                                     
      | Place copyright information at the top of every subsystem in design.
      mask prompts: none "No parameters"
      mask help: Place copyright information at the top of every subsystem in design.
      mask Display:
      | NxtrConf = 'Nexteer Confidential';
      | 
      | sys = bdroot; %handle for the current model ("system")
      | first = get_param(sys,'Created');
      | if(isempty(first))
      |     first = datestr(now,'yyyy');
      | else
      |     first = first(end-3:end);  %year is last four digits
      | end
      | 
      | last = get_param(sys,'LastModifiedDate');
      | if isempty(last)
      |     last = datestr(now,'yyyy');
      | else
      |     last = last(end-3:end);
      | end
      | 
      | if strcmp(first,last)
      |     fprintf('%s -- Copyright %s Nexteer',NxtrConf,first)
      | else
      |     fprintf('%s -- %s%s- %s Nexteer',NxtrConf,char(169),first,last)
      | end
  Count per uSec : Constant  Value=0.01
  Data Store Read1 : DataStoreRead  DataStoreName=SimnTi
  Data Type Conversion1 : DataTypeConversion  OutDataTypeStr=uint32
  Divide1 : Product  Inputs=**
  Divide2 : Product  Inputs=*/
  Max Counts : Constant  Value=2^32-1
  Product1 : Product
  Product2 : Product
  Rounding : Rounding
  Subtract1 : Sum  Inputs=+-
  uSec per Sec : Constant  Value=1000000
  RefTmr : Outport
  wires:
  Product2/1 -> Subtract1/2
  Subtract1/1 -> Data Type Conversion1/1
  Rounding/1 -> Product2/1
  Divide2/1 -> Rounding/1
  Max Counts/1 -> Divide2/2, Product2/2
  Divide1/1 -> Divide2/1, Subtract1/1
  Product1/1 -> Divide1/1
  Data Store Read1/1 -> Product1/1
  Count per uSec/1 -> Divide1/2
  uSec per Sec/1 -> Product1/2
  Data Type Conversion1/1 -> RefTmr/1

== system SF045A_HwAgSysArbn/HwAgSysArbn/HwAgSysArbnPer1/HwAgArbn/HwAgVelSeriCom/ChkCorrln/SetNtcPass/SetNtcPass ==
  NtcNr : Inport
  NtcStInfo : Inport  Port=2
  NtcSts : Inport  Port=3
  DebStep : Inport  Port=4
  SetNtcSts : Subsystem  RequirementInfo={} %GIDa_3e24807c_f7b6_481d_bf36_c20cd7c5d8b1  TreatAsAtomicUnit=on
      settings: RTWSystemCode=Inline
  wires:
  NtcNr/1 -> SetNtcSts/1(NtcNr)  "NtcNr"
  NtcSts/1 -> SetNtcSts/3(NtcSts)
  DebStep/1 -> SetNtcSts/4(DebStep)
  NtcStInfo/1 -> SetNtcSts/2(NtcStInfo)

== system SF045A_HwAgSysArbn/HwAgSysArbn/HwAgSysArbnPer1/HwAgArbn/HwAgVelSeriCom/SnsrlsDataToSerlCom/CorrlnStsFalse/CopyRight2 ==

== system SF045A_HwAgSysArbn/HwAgSysArbn/HwAgSysArbnPer1/HwAgArbn/HwAgVelSeriCom/SnsrlsDataToSerlCom/CorrlnStsTrue/CopyRight2 ==

== system SF045A_HwAgSysArbn/HwAgSysArbn/HwAgSysArbnPer1/HwAgArbn/HwAgVelSeriCom/SnsrlsDataToSerlCom/GetTiSpan100MicroSec32bit/CopyRight2 ==

== system SF045A_HwAgSysArbn/HwAgSysArbn/HwAgSysArbnPer1/HwAgArbn/HwAgVelSeriCom/SnsrlsDataToSerlCom/GetTiSpan100MicroSec32bit/No wrapping ==
  new : Inport
  ref : Inport  Port=2
  Action Port : ActionPort  ActionType=then
  CopyRight2 : Subsystem  Description=|  mask(Copyright Information){none=on}
      | Copyright info block.                                               
      |                                                                     
      | Place copyright information at the top of every subsystem in design.
      mask prompts: none "No parameters"
      mask help: Place copyright information at the top of every subsystem in design.
      mask Display:
      | NxtrConf = 'Nexteer Confidential';
      | 
      | sys = bdroot; %handle for the current model ("system")
      | first = get_param(sys,'Created');
      | if(isempty(first))
      |     first = datestr(now,'yyyy');
      | else
      |     first = first(end-3:end);  %year is last four digits
      | end
      | 
      | last = get_param(sys,'LastModifiedDate');
      | if isempty(last)
      |     last = datestr(now,'yyyy');
      | else
      |     last = last(end-3:end);
      | end
      | 
      | if strcmp(first,last)
      |     fprintf('%s -- Copyright %s Nexteer',NxtrConf,first)
      | else
      |     fprintf('%s -- %s%s- %s Nexteer',NxtrConf,char(169),first,last)
      | end
  Subtract1 : Sum  Inputs=+-
  Out1 : Outport
  wires:
  Subtract1/1 -> Out1/1
  new/1 -> Subtract1/1
  ref/1 -> Subtract1/2

== system SF045A_HwAgSysArbn/HwAgSysArbn/HwAgSysArbnPer1/HwAgArbn/HwAgVelSeriCom/SnsrlsDataToSerlCom/GetTiSpan100MicroSec32bit/Wrapping ==
  new : Inport
  ref : Inport  Port=2
  Action Port : ActionPort  ActionType=else
  CopyRight2 : Subsystem  Description=|  mask(Copyright Information){none=on}
      | Copyright info block.                                               
      |                                                                     
      | Place copyright information at the top of every subsystem in design.
      mask prompts: none "No parameters"
      mask help: Place copyright information at the top of every subsystem in design.
      mask Display:
      | NxtrConf = 'Nexteer Confidential';
      | 
      | sys = bdroot; %handle for the current model ("system")
      | first = get_param(sys,'Created');
      | if(isempty(first))
      |     first = datestr(now,'yyyy');
      | else
      |     first = first(end-3:end);  %year is last four digits
      | end
      | 
      | last = get_param(sys,'LastModifiedDate');
      | if isempty(last)
      |     last = datestr(now,'yyyy');
      | else
      |     last = last(end-3:end);
      | end
      | 
      | if strcmp(first,last)
      |     fprintf('%s -- Copyright %s Nexteer',NxtrConf,first)
      | else
      |     fprintf('%s -- %s%s- %s Nexteer',NxtrConf,char(169),first,last)
      | end
  Max Counts : Constant  Value=2^32-1  OutDataTypeStr=uint32
  Subtract1 : Sum  Inputs=+-+
  Out1 : Outport
  wires:
  Subtract1/1 -> Out1/1
  Max Counts/1 -> Subtract1/1
  ref/1 -> Subtract1/2
  new/1 -> Subtract1/3

== system SF045A_HwAgSysArbn/HwAgSysArbn/HwAgSysArbnPer1/HwAgArbn/TestHwAgSrcChg/ApplyRateLim/GetTiSpan100MicroSec32bit/CopyRight2 ==

== system SF045A_HwAgSysArbn/HwAgSysArbn/HwAgSysArbnPer1/HwAgArbn/TestHwAgSrcChg/ApplyRateLim/GetTiSpan100MicroSec32bit/No wrapping ==
  new : Inport
  ref : Inport  Port=2
  Action Port : ActionPort  ActionType=then
  CopyRight2 : Subsystem  Description=|  mask(Copyright Information){none=on}
      | Copyright info block.                                               
      |                                                                     
      | Place copyright information at the top of every subsystem in design.
      mask prompts: none "No parameters"
      mask help: Place copyright information at the top of every subsystem in design.
      mask Display:
      | NxtrConf = 'Nexteer Confidential';
      | 
      | sys = bdroot; %handle for the current model ("system")
      | first = get_param(sys,'Created');
      | if(isempty(first))
      |     first = datestr(now,'yyyy');
      | else
      |     first = first(end-3:end);  %year is last four digits
      | end
      | 
      | last = get_param(sys,'LastModifiedDate');
      | if isempty(last)
      |     last = datestr(now,'yyyy');
      | else
      |     last = last(end-3:end);
      | end
      | 
      | if strcmp(first,last)
      |     fprintf('%s -- Copyright %s Nexteer',NxtrConf,first)
      | else
      |     fprintf('%s -- %s%s- %s Nexteer',NxtrConf,char(169),first,last)
      | end
  Subtract1 : Sum  Inputs=+-
  Out1 : Outport
  wires:
  Subtract1/1 -> Out1/1
  new/1 -> Subtract1/1
  ref/1 -> Subtract1/2

== system SF045A_HwAgSysArbn/HwAgSysArbn/HwAgSysArbnPer1/HwAgArbn/TestHwAgSrcChg/ApplyRateLim/GetTiSpan100MicroSec32bit/Wrapping ==
  new : Inport
  ref : Inport  Port=2
  Action Port : ActionPort  ActionType=else
  CopyRight2 : Subsystem  Description=|  mask(Copyright Information){none=on}
      | Copyright info block.                                               
      |                                                                     
      | Place copyright information at the top of every subsystem in design.
      mask prompts: none "No parameters"
      mask help: Place copyright information at the top of every subsystem in design.
      mask Display:
      | NxtrConf = 'Nexteer Confidential';
      | 
      | sys = bdroot; %handle for the current model ("system")
      | first = get_param(sys,'Created');
      | if(isempty(first))
      |     first = datestr(now,'yyyy');
      | else
      |     first = first(end-3:end);  %year is last four digits
      | end
      | 
      | last = get_param(sys,'LastModifiedDate');
      | if isempty(last)
      |     last = datestr(now,'yyyy');
      | else
      |     last = last(end-3:end);
      | end
      | 
      | if strcmp(first,last)
      |     fprintf('%s -- Copyright %s Nexteer',NxtrConf,first)
      | else
      |     fprintf('%s -- %s%s- %s Nexteer',NxtrConf,char(169),first,last)
      | end
  Max Counts : Constant  Value=2^32-1  OutDataTypeStr=uint32
  Subtract1 : Sum  Inputs=+-+
  Out1 : Outport
  wires:
  Subtract1/1 -> Out1/1
  Max Counts/1 -> Subtract1/1
  ref/1 -> Subtract1/2
  new/1 -> Subtract1/3

== system SF045A_HwAgSysArbn/HwAgSysArbn/HwAgSysArbnPer1/HwAgArbn/TestHwAgSrcChg/ApplyRateLim/Pass/CopyRight2 ==

== system SF045A_HwAgSysArbn/HwAgSysArbn/HwAgSysArbnPer1/HwAgArbn/TestHwAgSrcChg/ApplyRateLim/RetainHwAgConf/CopyRight2 ==

== system SF045A_HwAgSysArbn/HwAgSysArbn/HwAgSysArbnPer1/HwAgArbn/TestHwAgSrcChg/SetSlewRate/GetRefTmr100MicroSec32bit/CopyRight2 ==
